simulink model "finalsim_version_2018"  (R2018a)
settings: Solver=VariableStepAuto  StartTime=0.0  StopTime=4  RelTol=1e-3
values from neighbouring files (symbols this model uses):
  Ts = 0.017    [Final_Control_Automatico_plain.m]
undefined symbols (not defined in the file or in its folder): denC, denCd, denG, denH, numC, numCd, numG, numH
libraries: simulink x2, powerlib_meascontrol x1
settings Model: Creator=Trini  LastModifiedBy=Trini

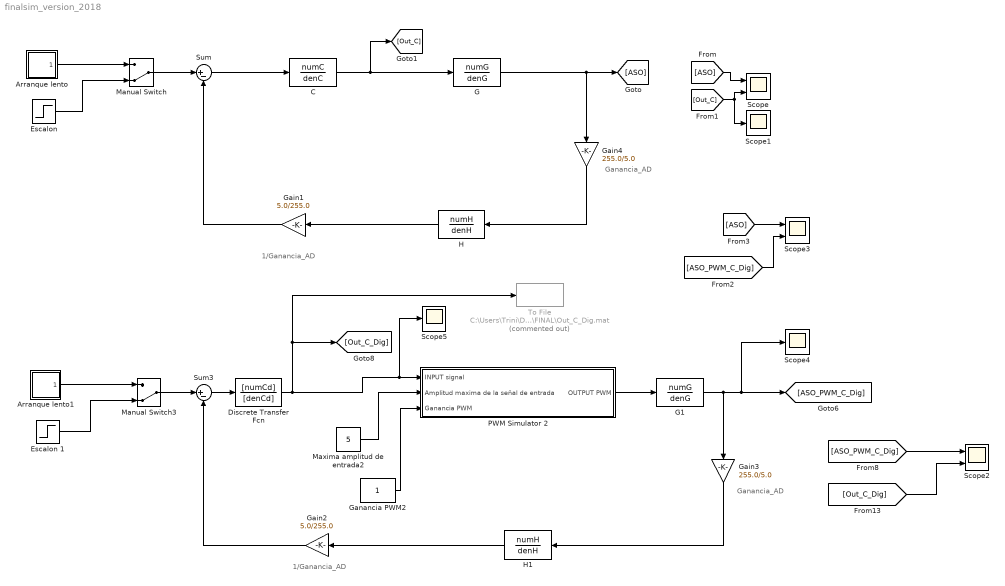
== system finalsim_version_2018 ==
  note: Ganancia_AD
  note: 1/Ganancia_AD
  note: Ganancia_AD
  note: 1/Ganancia_AD
  Arranque lento : Subsystem
  Arranque lento1 : Subsystem
  "C " : TransferFcn  Numerator=numC  Denominator=denC
  Discrete Transfer Fcn : DiscreteTransferFcn  Numerator=[numCd]  Denominator=[denCd]  SampleTime=Ts
  "Escalon " : Step  Time=0.5  SampleTime=0
  Escalon 1 : Step  Time=0.5  SampleTime=0
  G : TransferFcn  Numerator=numG  Denominator=denG
  G1 : TransferFcn  Numerator=numG  Denominator=denG
  Gain1 : Gain  Gain=5.0/255.0
  Gain2 : Gain  Gain=5.0/255.0
  Gain3 : Gain  Gain=255.0/5.0
  Gain4 : Gain  Gain=255.0/5.0
  Ganancia PWM2 : Constant
  H : TransferFcn  Numerator=numH  Denominator=denH
  H1 : TransferFcn  Numerator=numH  Denominator=denH
  Manual Switch : ManualSwitch  CurrentSetting=0
  Manual Switch3 : ManualSwitch  CurrentSetting=0
  Maxima amplitud de entrada2 : Constant  Value=5
  PWM Simulator 2 : Subsystem
  Scope : Scope  NumInputPorts=2
  Scope1 : Scope
  Scope2 : Scope  NumInputPorts=2
  Scope3 : Scope  NumInputPorts=2
  Scope4 : Scope
  Scope5 : Scope
  Sum : Sum  Inputs=|+-
  Sum3 : Sum  Inputs=|+-
  To File : ToFile  Commented=on  Filename=C:\Users\Trini\Documents\UCA\5° Año\Segundo Cuatrimestre\Control Automatico\FINAL\Out_C_Dig.mat  MatrixName=Out_C_Dig
  wires:
  Arranque lento/1(Out1) -> Manual Switch/1
  "C "/1 -> G/1, [Out_C]
  Sum/1 -> "C "/1
  G/1 -> Gain4/1, [ASO]
  Gain4/1 -> H/1
  H/1 -> Gain1/1
  Gain1/1 -> Sum/2
  "Escalon "/1 -> Manual Switch/2
  [ASO] -> Scope/1
  [Out_C] -> Scope1/1, Scope/2
  Manual Switch/1 -> Sum/1
  Gain2/1 -> Sum3/2
  Discrete Transfer Fcn/1 -> To File/1, [Out_C_Dig], Scope5/1, PWM Simulator 2/1(INPUT signal)
  [ASO_PWM_C_Dig] -> Scope2/1
  Sum3/1 -> Discrete Transfer Fcn/1
  Maxima amplitud de entrada2/1 -> PWM Simulator 2/2("Amplitud maxima de la señal de entrada ")
  G1/1 -> Scope4/1, [ASO_PWM_C_Dig], Gain3/1
  Ganancia PWM2/1 -> PWM Simulator 2/3("Ganancia PWM ")
  Manual Switch3/1 -> Sum3/1
  H1/1 -> Gain2/1
  PWM Simulator 2/1(OUTPUT PWM) -> G1/1
  Gain3/1 -> H1/1
  Arranque lento1/1(Out1) -> Manual Switch3/1
  Escalon 1/1 -> Manual Switch3/2
  [Out_C_Dig] -> Scope2/2
  [ASO_PWM_C_Dig] -> Scope3/2
  [ASO] -> Scope3/1

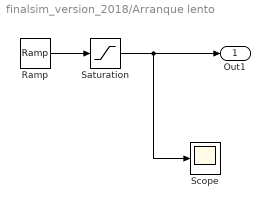
== system finalsim_version_2018/Arranque lento ==
  Ramp : simulink/Sources/Ramp  slope=120  start=1  InitialOutput=0
  Saturation : Saturate  UpperLimit=1  LowerLimit=0
  Scope : Scope
  Out1 : Outport
  wires:
  Ramp/1 -> Saturation/1
  Saturation/1 -> Scope/1, Out1/1

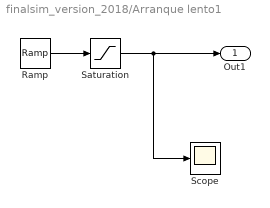
== system finalsim_version_2018/Arranque lento1 ==
  Ramp : simulink/Sources/Ramp  slope=120  start=1  InitialOutput=0
  Saturation : Saturate  UpperLimit=51  LowerLimit=0
  Scope : Scope
  Out1 : Outport
  wires:
  Ramp/1 -> Saturation/1
  Saturation/1 -> Scope/1, Out1/1

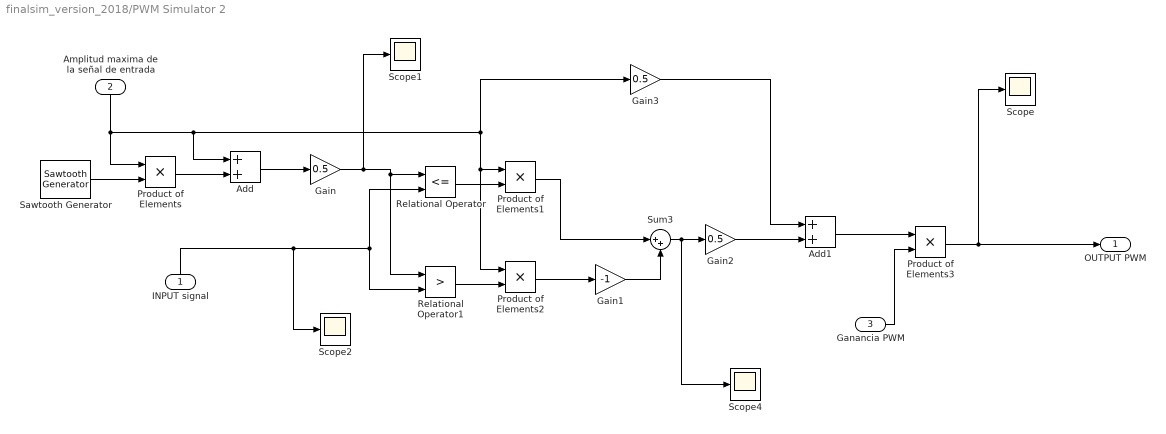
== system finalsim_version_2018/PWM Simulator 2 ==
  INPUT signal : Inport
  "Amplitud maxima de la señal de entrada " : Inport  Port=2
  "Ganancia PWM " : Inport  Port=3
  Add : Sum
  Add1 : Sum
  Gain : Gain  Gain=0.5
  Gain1 : Gain  Gain=-1
  Gain2 : Gain  Gain=0.5
  Gain3 : Gain  Gain=0.5
  Product of Elements{,1..3} (4 alike) : Product  Inputs=**
  Relational Operator : RelationalOperator  Operator=<=  OutDataTypeStr=boolean  RndMeth=Nearest
  Relational Operator1 : RelationalOperator  Operator=>  OutDataTypeStr=boolean  RndMeth=Nearest
  Sawtooth Generator : powerlib_meascontrol/Pulse & Signal Generators/Sawtooth Generator  Freq=200  Phase=180  Ts=0
      settings: SourceProductName=Simscape Power Systems
  Scope{,1..2,4} (4 alike) : Scope
  Sum3 : Sum  Inputs=|++
  OUTPUT PWM : Outport
  wires:
  "Amplitud maxima de la señal de entrada "/1 -> Add/1, Product of Elements2/1, Product of Elements1/1, Gain3/1, Product of Elements/1
  Relational Operator/1 -> Product of Elements1/2
  Relational Operator1/1 -> Product of Elements2/2
  Product of Elements1/1 -> Sum3/1
  Product of Elements2/1 -> Gain1/1
  Gain1/1 -> Sum3/2
  Sum3/1 -> Scope4/1, Gain2/1
  "Ganancia PWM "/1 -> Product of Elements3/2
  INPUT signal/1 -> Scope2/1, Relational Operator1/2, Relational Operator/2
  Sawtooth Generator/1 -> Product of Elements/2
  Add/1 -> Gain/1
  Product of Elements/1 -> Add/2
  Gain/1 -> Scope1/1, Relational Operator1/1, Relational Operator/1
  Add1/1 -> Product of Elements3/1
  Gain2/1 -> Add1/2
  Gain3/1 -> Add1/1
  Product of Elements3/1 -> OUTPUT PWM/1, Scope/1
